simulink model "Practica_3_Simulink"  (R2024b)
settings: Solver=VariableStepAuto  StartTime=0.0  StopTime=10  RelTol=1e-3
InitFcn:
  | m1 = 290;   % Masa 1
  | m2 = 59;    % Masa 2
  | k1 = 16182; % Constante del resorte 1
  | k2 = 19000; % Constante del resorte 2
  | b1 = 1000;  % Coeficiente de amortiguamiento
  | f = 0;      % Fuerza externa
settings Model: Creator=RAM  LastModifiedBy=RAM

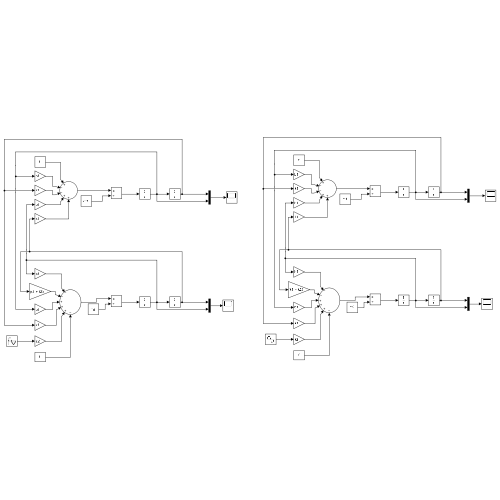
[thumbnail: Simulink's stored preview of the top-level diagram]
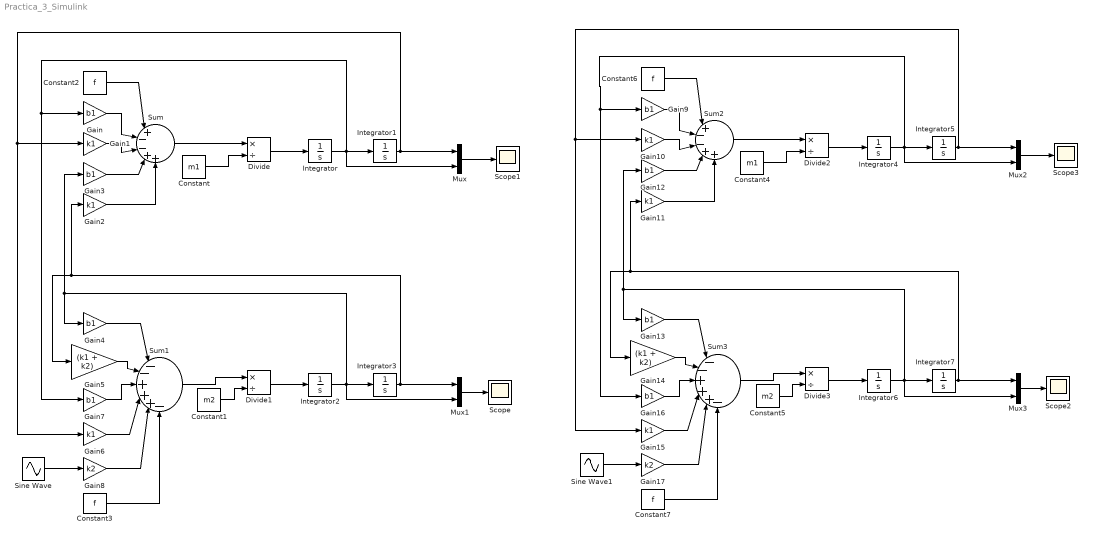
== system Practica_3_Simulink ==
  Constant : Constant  Value=m1
  Constant1 : Constant  Value=m2
  Constant{2..3,6..7} (4 alike) : Constant  Value=f
  Constant4 : Constant  Value=m1
  Constant5 : Constant  Value=m2
  Divide{,1..3} (4 alike) : Product  Inputs=*/
  Gain{,3..4,7,9,12..13,16} (8 alike) : Gain  Gain=b1
  Gain{1..2,6,10..11,15} (6 alike) : Gain  Gain=k1
  Gain14 : Gain  Gain=(k1 + k2)
  Gain17 : Gain  Gain=k2
  Gain5 : Gain  Gain=(k1 + k2)
  Gain8 : Gain  Gain=k2
  Integrator{,1..7} (8 alike) : Integrator
  Mux{,1..3} (4 alike) : Mux  Inputs=2
  Scope{,1..3} (4 alike) : Scope
  Sine Wave : Sin  Amplitude=0.05  Frequency=0.5* pi  SampleTime=0
  Sine Wave1 : Sin  Amplitude=0.05  Frequency=20* pi  SampleTime=0
  Sum : Sum  Inputs=|+--++
  Sum1 : Sum  Inputs=|--+++-
  Sum2 : Sum  Inputs=|+--++
  Sum3 : Sum  Inputs=|--+++-
  wires:
  Sum/1 -> Divide/1
  Constant/1 -> Divide/2
  Divide/1 -> Integrator/1
  Integrator/1 -> Mux/2, Gain7/1, Gain/1, Integrator1/1
  Gain/1 -> Sum/2
  Gain1/1 -> Sum/3
  Gain3/1 -> Sum/4
  Gain2/1 -> Sum/5
  Integrator1/1 -> Gain6/1, Gain1/1, Mux/1
  Integrator3/1 -> Mux1/1, Gain2/1, Gain5/1
  Gain6/1 -> Sum1/4
  Gain7/1 -> Sum1/3
  Gain5/1 -> Sum1/2
  Gain4/1 -> Sum1/1
  Integrator2/1 -> Integrator3/1, Gain3/1, Gain4/1, Mux1/2
  Divide1/1 -> Integrator2/1
  Constant1/1 -> Divide1/2
  Sum1/1 -> Divide1/1
  Constant2/1 -> Sum/1
  Mux1/1 -> Scope/1
  Mux/1 -> Scope1/1
  Sine Wave/1 -> Gain8/1
  Gain8/1 -> Sum1/5
  Constant3/1 -> Sum1/6
  Constant7/1 -> Sum3/6
  Gain17/1 -> Sum3/5
  Sine Wave1/1 -> Gain17/1
  Mux2/1 -> Scope3/1
  Mux3/1 -> Scope2/1
  Constant6/1 -> Sum2/1
  Sum3/1 -> Divide3/1
  Constant5/1 -> Divide3/2
  Divide3/1 -> Integrator6/1
  Integrator6/1 -> Mux3/2, Gain13/1, Gain12/1, Integrator7/1
  Gain13/1 -> Sum3/1
  Gain14/1 -> Sum3/2
  Gain16/1 -> Sum3/3
  Gain15/1 -> Sum3/4
  Integrator7/1 -> Gain14/1, Gain11/1, Mux3/1
  Integrator5/1 -> Mux2/1, Gain10/1, Gain15/1
  Gain11/1 -> Sum2/5
  Gain12/1 -> Sum2/4
  Gain10/1 -> Sum2/3
  Gain9/1 -> Sum2/2
  Integrator4/1 -> Integrator5/1, Gain9/1, Gain16/1, Mux2/2
  Divide2/1 -> Integrator4/1
  Constant4/1 -> Divide2/2
  Sum2/1 -> Divide2/1
